simulink model "pdgrav"  (R2020b)
settings: Solver=VariableStepAuto  StartTime=0.0  StopTime=15  RelTol=1e-3
values from neighbouring files (symbols this model uses):
  g = 9.81    [run_sim_asn5q1.m]    (also in run_sim_asn5q1c.m)
  l1 = 1    [run_sim_asn5q1.m]    (also in run_sim_asn5q1c.m)
  l2 = 1    [run_sim_asn5q1.m]    (also in run_sim_asn5q1c.m)
  m1 = 1    [run_sim_asn5q1.m]    (also in run_sim_asn5q1c.m)
  m2 = 1    [run_sim_asn5q1.m]    (also in run_sim_asn5q1c.m)
  x_0 = x_0_in    [run_sim_asn5q1.m]    (also in run_sim_asn5q1c.m)
undefined symbols (not defined in the file or in its folder): Kp, Kv, q_d
settings Model: Creator=zhich  LastModifiedBy=zhich

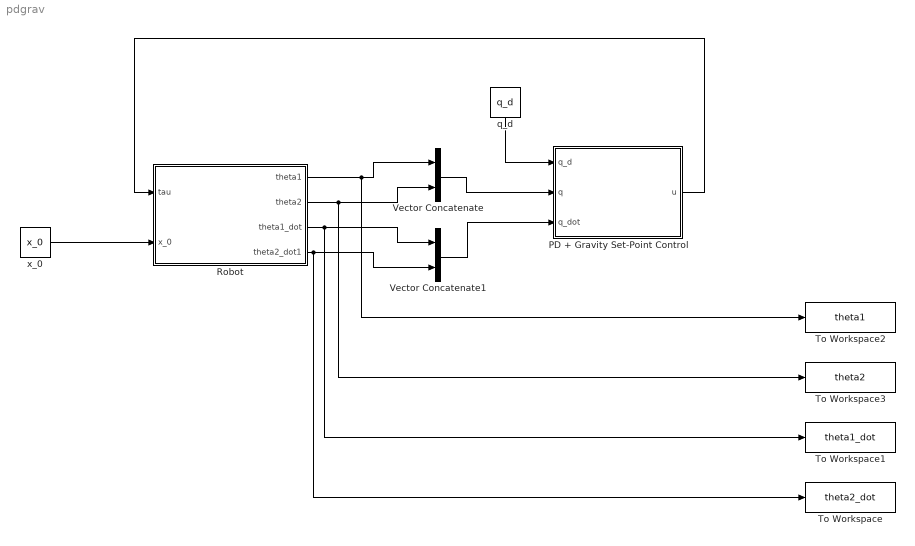
== system pdgrav ==
  PD + Gravity Set-Point Control : Subsystem
  Robot : Subsystem
  To Workspace : ToWorkspace  VariableName=theta2_dot  SaveFormat=Timeseries  SampleTime=-1
  To Workspace1 : ToWorkspace  VariableName=theta1_dot  SaveFormat=Timeseries  SampleTime=-1
  To Workspace2 : ToWorkspace  VariableName=theta1  SaveFormat=Timeseries  SampleTime=-1
  To Workspace3 : ToWorkspace  VariableName=theta2  SaveFormat=Timeseries  SampleTime=-1
  Vector Concatenate : Concatenate
  Vector Concatenate1 : Concatenate
  q_d : Constant  Value=q_d
  x_0 : Constant  Value=x_0
  wires:
  x_0/1 -> Robot/2(x_0)
  Robot/1(theta1) -> To Workspace2/1, Vector Concatenate/1
  Robot/2(theta2) -> Vector Concatenate/2, To Workspace3/1
  Vector Concatenate/1 -> PD + Gravity Set-Point Control/2(q)
  PD + Gravity Set-Point Control/1(u) -> Robot/1(tau)
  q_d/1 -> PD + Gravity Set-Point Control/1(q_d)
  Robot/4(theta2_dot1) -> Vector Concatenate1/2, To Workspace/1
  Robot/3(theta1_dot) -> Vector Concatenate1/1, To Workspace1/1
  Vector Concatenate1/1 -> PD + Gravity Set-Point Control/3(q_dot)

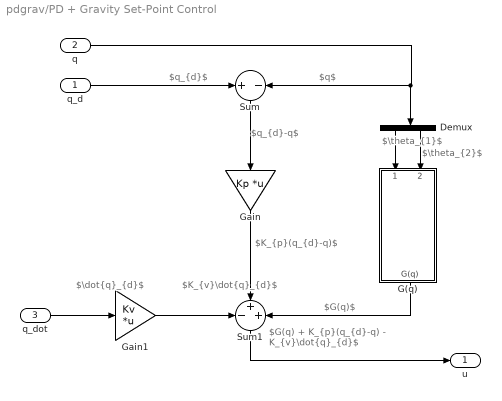
== system pdgrav/PD + Gravity Set-Point Control ==
  note: $\theta_{1}$
  note: $\theta_{2}$
  note: $G(q)$
  note: $q_{d}$
  note: $q$
  note: $q_{d}-q$
  note: $K_{p}(q_{d}-q)$
  note: $\dot{q}_{d}$
  note: $K_{v}\dot{q}_{d}$
  note: $G(q) + K_{p}(q_{d}-q) - K_{v}\dot{q}_{d}$
  q_d : Inport
  q : Inport  Port=2
  q_dot : Inport  Port=3
  Demux : Demux  Outputs=2
  G(q) : Subsystem
  Gain : Gain  Gain=Kp  Multiplication=Matrix(K*u)
  Gain1 : Gain  Gain=Kv  Multiplication=Matrix(K*u)
  Sum : Sum  Inputs=+|-
  Sum1 : Sum  Inputs=-++
  u : Outport
  wires:
  q_d/1 -> Sum/1
  q/1 -> Sum/2, Demux/1
  Demux/1 -> G(q)/1(theta1)
  Demux/2 -> G(q)/2(theta2)
  G(q)/1(G(q)) -> Sum1/3
  Sum/1 -> Gain/1
  q_dot/1 -> Gain1/1
  Gain1/1 -> Sum1/1
  Gain/1 -> Sum1/2
  Sum1/1 -> u/1

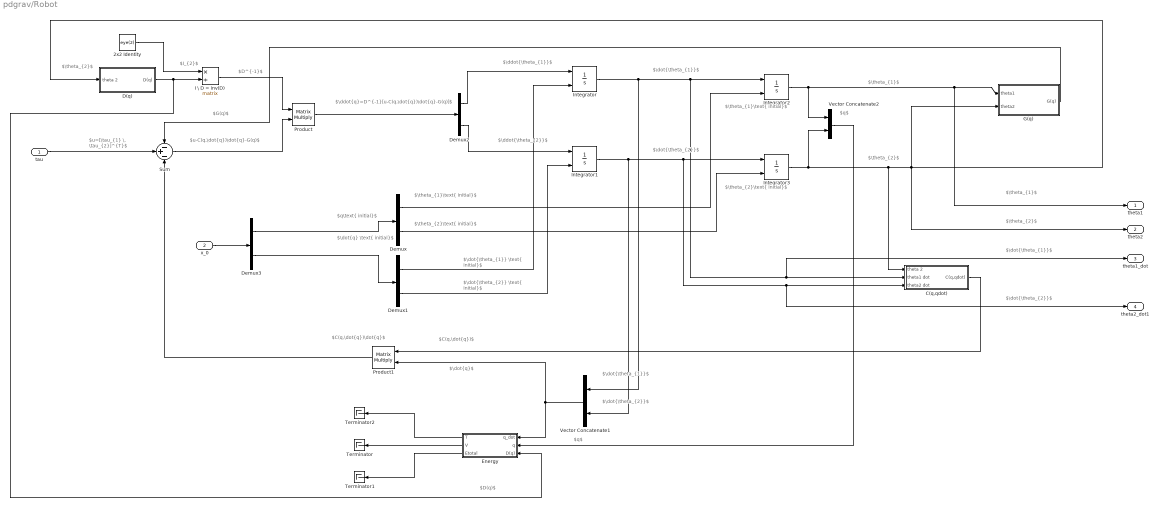
== system pdgrav/Robot ==
  note: $\dot{\theta_{2}}$
  note: $q$
  note: $D^{-1}$
  note: $\theta_{1}$
  note: $\theta_{2}\text{ initial}$
  note: $\dot{\theta_{1}}$
  note: $\theta_{2}$
  note: $q$
  note: $\dot{\theta_{1}}$
  note: $D(q)$
  note: $\ddot{\theta_{2}}$
  note: $\dot{\theta_{1}}$
  note: $\dot{q} \text{ initial}$
  note: $\theta_{2}$
  note: $I_{2}$
  note: $\theta_{1}\text{ initial}$
  note: $\dot{q}$
  note: $\theta_{2}$
  note: $\ddot{q}=D^{-1}[u-C(q,\dot{q})\dot{q}-G(q)]$
  note: $\dot{\theta_{1}} \text{ initial}$
  note: $u=[\tau_{1} \, \tau_{2}]^{T}$
  note: $G(q)$
  note: $\theta_{1}\text{ initial}$
  note: $\dot{\theta_{2}} \text{ initial}$
  note: $\dot{\theta_{2}}$
  note: $\theta_{1}$
  note: $\theta_{2}\text{ initial}$
  note: $q\text{ initial}$
  note: $C(q,\dot{q})\dot{q}$
  note: $u-C(q,\dot{q})\dot{q}-G(q)$
  note: $\dot{\theta_{2}}$
  note: $\ddot{\theta_{1}}$
  note: $C(q,\dot{q})$
  tau : Inport
  x_0 : Inport  Port=2
  2x2 Identity : Constant  Value=eye(2)
  C(q,qdot) : Subsystem
  D(q) : Subsystem
  Demux{,1..3} (4 alike) : Demux  Outputs=2
  Energy : Subsystem
  G(q) : Subsystem
  I \ D = inv(D) : Product  Inputs=*/  Multiplication=Matrix(*)
  Integrator{,1..3} (4 alike) : Integrator  InitialConditionSource=external
  Product : Product  Multiplication=Matrix(*)
  Product1 : Product  Multiplication=Matrix(*)
  Sum : Sum  Inputs=-+-
  Terminator : Terminator
  Terminator1 : Terminator
  Terminator2 : Terminator
  Vector Concatenate1 : Concatenate
  Vector Concatenate2 : Concatenate
  theta1 : Outport
  theta2 : Outport  Port=2
  theta1_dot : Outport  Port=3
  theta2_dot1 : Outport  Port=4
  wires:
  Energy/2(V) -> Terminator/1
  Demux3/2 -> Demux1/1
  tau/1 -> Sum/2
  Demux2/2 -> Integrator1/1
  Integrator/1 -> theta1_dot/1, C(q,qdot)/2(theta1 dot), Integrator2/1, Vector Concatenate1/1
  G(q)/1(G(q)) -> Sum/1
  Energy/3(Etotal) -> Terminator1/1
  Integrator3/1 -> Vector Concatenate2/2, theta2/1, D(q)/1(theta 2), G(q)/2(theta2), C(q,qdot)/1(theta 2)
  x_0/1 -> Demux3/1
  Vector Concatenate1/1 -> Product1/2, Energy/1(q_dot)
  Vector Concatenate2/1 -> Energy/2(q)
  Energy/1(T) -> Terminator2/1
  Integrator2/1 -> Vector Concatenate2/1, theta1/1, G(q)/1(theta1)
  Demux/2 -> Integrator3/2
  Demux1/2 -> Integrator1/2
  2x2 Identity/1 -> I \ D = inv(D)/1
  Demux1/1 -> Integrator/2
  I \ D = inv(D)/1 -> Product/1
  D(q)/1(D(q)) -> Energy/3(D(q)), I \ D = inv(D)/2
  Demux3/1 -> Demux/1
  Sum/1 -> Product/2
  Demux2/1 -> Integrator/1
  Product1/1 -> Sum/3
  Demux/1 -> Integrator2/2
  Integrator1/1 -> theta2_dot1/1, C(q,qdot)/3(theta2 dot), Integrator3/1, Vector Concatenate1/2
  C(q,qdot)/1(C(q,qdot)) -> Product1/1
  Product/1 -> Demux2/1

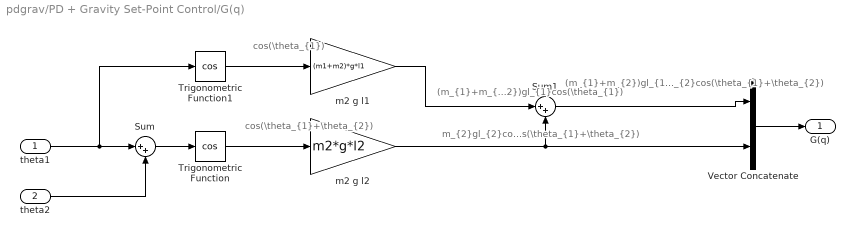
== system pdgrav/PD + Gravity Set-Point Control/G(q) ==
  note: cos(\theta_{1})
  note: (m_{1}+m_{2})gl_{1}cos(\theta_{1})+m_{2}gl_{2}cos(\theta_{1}+\theta_{2})
  note: (m_{1}+m_{2})gl_{1}cos(\theta_{1})
  note: m_{2}gl_{2}cos(\theta_{1}+\theta_{2})
  note: cos(\theta_{1}+\theta_{2})
  theta1 : Inport
  theta2 : Inport  Port=2
  Sum : Sum  Inputs=|++
  Sum1 : Sum  Inputs=|++
  Trigonometric Function : Trigonometry  Operator=cos
  Trigonometric Function1 : Trigonometry  Operator=cos
  Vector Concatenate : Concatenate
  m2 g l1 : Gain  Gain=(m1+m2)*g*l1
  m2 g l2 : Gain  Gain=m2*g*l2
  G(q) : Outport
  wires:
  theta1/1 -> Trigonometric Function1/1, Sum/1
  theta2/1 -> Sum/2
  Sum/1 -> Trigonometric Function/1
  Trigonometric Function/1 -> m2 g l2/1
  Vector Concatenate/1 -> G(q)/1
  m2 g l2/1 -> Sum1/2, Vector Concatenate/2
  Trigonometric Function1/1 -> m2 g l1/1
  m2 g l1/1 -> Sum1/1
  Sum1/1 -> Vector Concatenate/1

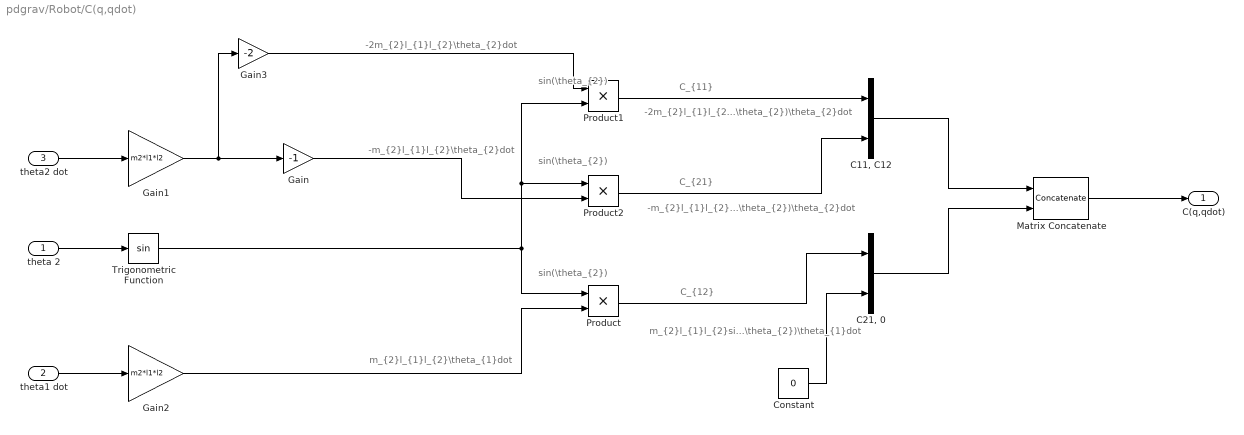
== system pdgrav/Robot/C(q,qdot) ==
  note: C_{21}
  note: -m_{2}l_{1}l_{2}\theta_{2}dot
  note: sin(\theta_{2})
  note: sin(\theta_{2})
  note: sin(\theta_{2})
  note: -2m_{2}l_{1}l_{2}\theta_{2}dot
  note: m_{2}l_{1}l_{2}\theta_{1}dot
  note: -m_{2}l_{1}l_{2}sin(\theta_{2})\theta_{2}dot
  note: C_{12}
  note: -2m_{2}l_{1}l_{2}sin(\theta_{2})\theta_{2}dot
  note: m_{2}l_{1}l_{2}sin(\theta_{2})\theta_{1}dot
  note: C_{11}
  theta 2 : Inport
  theta1 dot : Inport  Port=2
  theta2 dot : Inport  Port=3
  "C11, C12" : Concatenate
  "C21, 0" : Concatenate
  Constant : Constant  Value=0
  Gain : Gain  Gain=-1
  Gain1 : Gain  Gain=m2*l1*l2
  Gain2 : Gain  Gain=m2*l1*l2
  Gain3 : Gain  Gain=-2
  Matrix Concatenate : Concatenate  Mode=Multidimensional array  ConcatenateDimension=2
  Product : Product
  Product1 : Product
  Product2 : Product
  Trigonometric Function : Trigonometry
  C(q,qdot) : Outport
  wires:
  theta 2/1 -> Trigonometric Function/1
  theta1 dot/1 -> Gain2/1
  theta2 dot/1 -> Gain1/1
  Gain2/1 -> Product/2
  Trigonometric Function/1 -> Product/1, Product1/2, Product2/1
  Product/1 -> "C21, 0"/1
  Gain1/1 -> Gain3/1, Gain/1
  Gain/1 -> Product2/2
  Gain3/1 -> Product1/1
  Product2/1 -> "C11, C12"/2
  Matrix Concatenate/1 -> C(q,qdot)/1
  Product1/1 -> "C11, C12"/1
  "C11, C12"/1 -> Matrix Concatenate/1
  Constant/1 -> "C21, 0"/2
  "C21, 0"/1 -> Matrix Concatenate/2

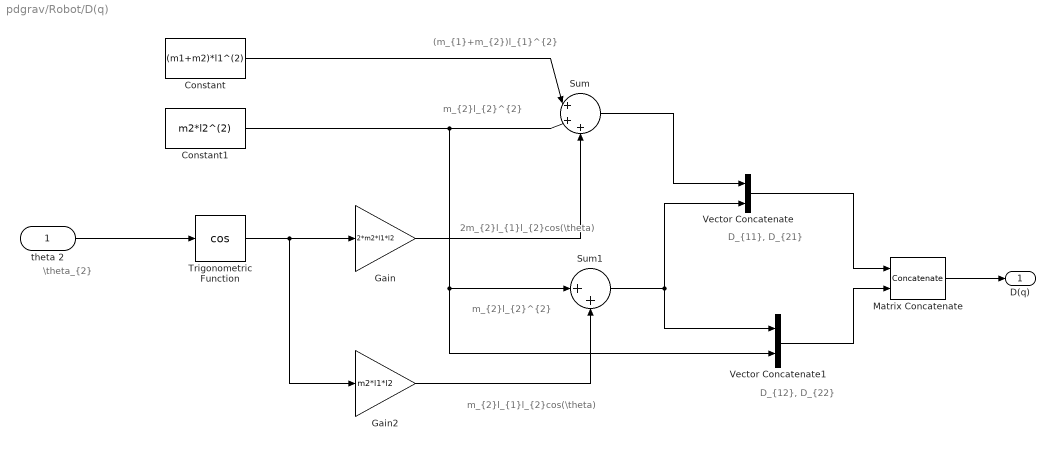
== system pdgrav/Robot/D(q) ==
  note: D_{12}, D_{22}
  note: D_{11}, D_{21}
  note: (m_{1}+m_{2})l_{1}^{2}
  note: \theta_{2}
  note: m_{2}l_{2}^{2}
  note: 2m_{2}l_{1}l_{2}cos(\theta)
  note: m_{2}l_{2}^{2}
  note: m_{2}l_{1}l_{2}cos(\theta)
  theta 2 : Inport
  Constant : Constant  Value=(m1+m2)*l1^(2)
  Constant1 : Constant  Value=m2*l2^(2)
  Gain : Gain  Gain=2*m2*l1*l2
  Gain2 : Gain  Gain=m2*l1*l2
  Matrix Concatenate : Concatenate  Mode=Multidimensional array  ConcatenateDimension=2
  Sum : Sum  Inputs=|+++
  Sum1 : Sum  Inputs=|++
  Trigonometric Function : Trigonometry  Operator=cos
  Vector Concatenate : Concatenate
  Vector Concatenate1 : Concatenate
  D(q) : Outport
  wires:
  theta 2/1 -> Trigonometric Function/1
  Trigonometric Function/1 -> Gain/1, Gain2/1
  Vector Concatenate/1 -> Matrix Concatenate/1
  Matrix Concatenate/1 -> D(q)/1
  Sum/1 -> Vector Concatenate/1
  Gain/1 -> Sum/3
  Constant1/1 -> Vector Concatenate1/2, Sum1/1, Sum/2
  Gain2/1 -> Sum1/2
  Sum1/1 -> Vector Concatenate1/1, Vector Concatenate/2
  Constant/1 -> Sum/1
  Vector Concatenate1/1 -> Matrix Concatenate/2

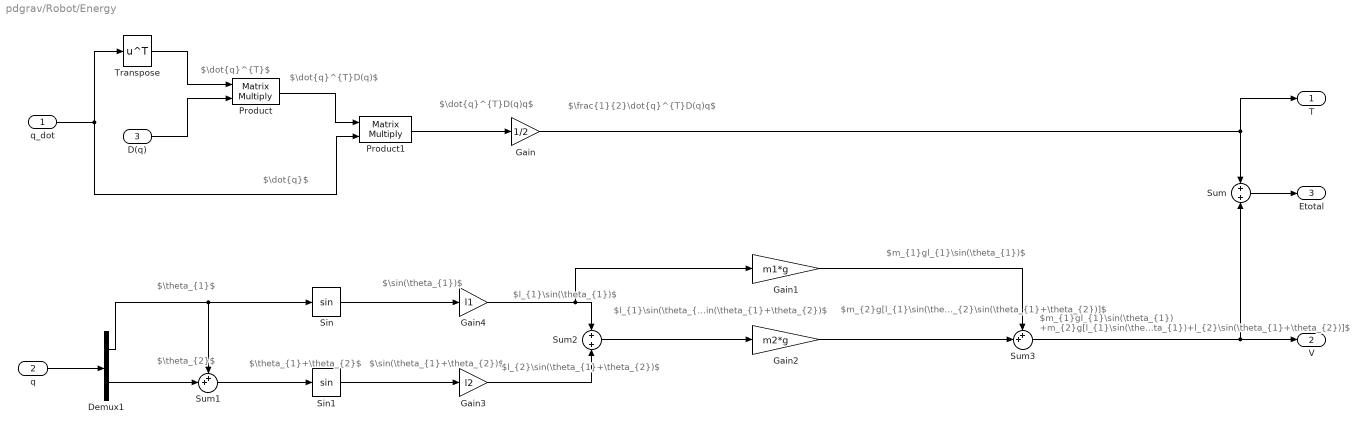
== system pdgrav/Robot/Energy ==
  note: $\dot{q}^{T}$
  note: $\dot{q}^{T}D(q)$
  note: $\dot{q}$
  note: $\dot{q}^{T}D(q)q$
  note: $\frac{1}{2}\dot{q}^{T}D(q)q$
  note: $\theta_{1}$
  note: $\theta_{2}$
  note: $\theta_{1}+\theta_{2}$
  note: $\sin(\theta_{1}+\theta_{2})$
  note: $\sin(\theta_{1})$
  note: $l_{1}\sin(\theta_{1})$
  note: $l_{2}\sin(\theta_{1}+\theta_{2})$
  note: $l_{1}\sin(\theta_{1})+l_{2}\sin(\theta_{1}+\theta_{2})$
  note: $m_{2}g[l_{1}\sin(\theta_{1})+l_{2}\sin(\theta_{1}+\theta_{2})]$
  note: $m_{1}gl_{1}\sin(\theta_{1})$
  note: $m_{1}gl_{1}\sin(\theta_{1}) +m_{2}g[l_{1}\sin(\theta_{1})+l_{2}\sin(\theta_{1}+\theta_{2})]$
  q_dot : Inport
  q : Inport  Port=2
  D(q) : Inport  Port=3
  Demux1 : Demux  Outputs=2
  Gain : Gain  Gain=1/2
  Gain1 : Gain  Gain=m1*g
  Gain2 : Gain  Gain=m2*g
  Gain3 : Gain  Gain=l2
  Gain4 : Gain  Gain=l1
  Product : Product  Multiplication=Matrix(*)
  Product1 : Product  Multiplication=Matrix(*)
  Sin : Trigonometry
  Sin1 : Trigonometry
  Sum : Sum
  Sum1 : Sum  Inputs=++|
  Sum2 : Sum
  Sum3 : Sum  Inputs=++|
  Transpose : Math  Operator=transpose  SaturateOnIntegerOverflow=on
  T : Outport
  V : Outport  Port=2
  Etotal : Outport  Port=3
  wires:
  q_dot/1 -> Transpose/1, Product1/2
  q/1 -> Demux1/1
  Transpose/1 -> Product/1
  D(q)/1 -> Product/2
  Product/1 -> Product1/1
  Product1/1 -> Gain/1
  Gain/1 -> T/1, Sum/1
  Sum/1 -> Etotal/1
  Demux1/1 -> Sin/1, Sum1/1
  Demux1/2 -> Sum1/2
  Sum1/1 -> Sin1/1
  Sin/1 -> Gain4/1
  Sin1/1 -> Gain3/1
  Gain4/1 -> Gain1/1, Sum2/1
  Gain3/1 -> Sum2/2
  Sum2/1 -> Gain2/1
  Gain2/1 -> Sum3/2
  Gain1/1 -> Sum3/1
  Sum3/1 -> Sum/2, V/1

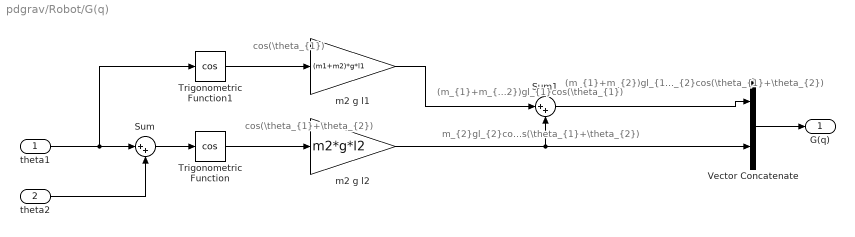
== system pdgrav/Robot/G(q) ==
  note: cos(\theta_{1})
  note: (m_{1}+m_{2})gl_{1}cos(\theta_{1})+m_{2}gl_{2}cos(\theta_{1}+\theta_{2})
  note: (m_{1}+m_{2})gl_{1}cos(\theta_{1})
  note: m_{2}gl_{2}cos(\theta_{1}+\theta_{2})
  note: cos(\theta_{1}+\theta_{2})
  theta1 : Inport
  theta2 : Inport  Port=2
  Sum : Sum  Inputs=|++
  Sum1 : Sum  Inputs=|++
  Trigonometric Function : Trigonometry  Operator=cos
  Trigonometric Function1 : Trigonometry  Operator=cos
  Vector Concatenate : Concatenate
  m2 g l1 : Gain  Gain=(m1+m2)*g*l1
  m2 g l2 : Gain  Gain=m2*g*l2
  G(q) : Outport
  wires:
  theta1/1 -> Trigonometric Function1/1, Sum/1
  theta2/1 -> Sum/2
  Sum/1 -> Trigonometric Function/1
  Trigonometric Function/1 -> m2 g l2/1
  Vector Concatenate/1 -> G(q)/1
  m2 g l2/1 -> Sum1/2, Vector Concatenate/2
  Trigonometric Function1/1 -> m2 g l1/1
  m2 g l1/1 -> Sum1/1
  Sum1/1 -> Vector Concatenate/1
